simulink model "ThermalBehaviour_simulink"  (R2022a)
settings: Solver=FixedStepAuto  StartTime=0.0  StopTime=10.0  FixedStep=1  RelTol=1e-3
settings Model: Creator=Anupp  LastModifiedBy=Anupp

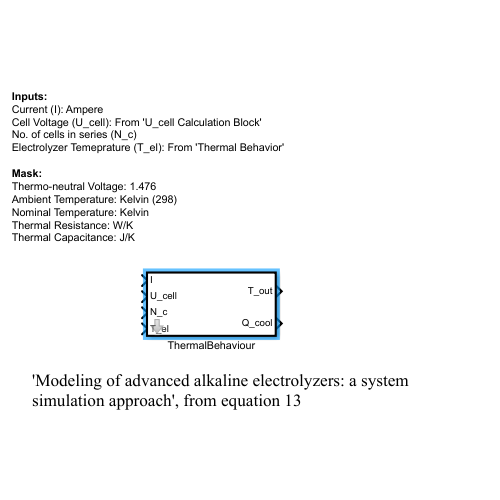
[thumbnail: Simulink's stored preview of the top-level diagram]
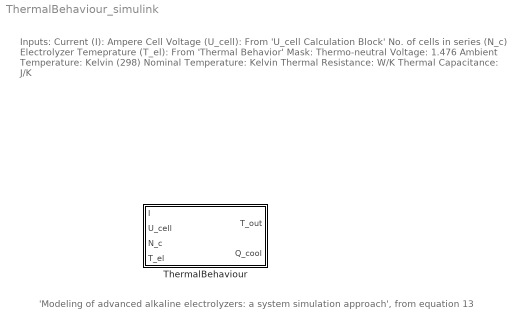
== system ThermalBehaviour_simulink ==
  note: Inputs:
      | Current (I): Ampere
      | Cell Voltage (U_cell): From 'U_cell Calculation Block'
      | No. of cells in series (N_c)
      | Electrolyzer Temeprature (T_el): From 'Thermal Behavior'
      |
      | Mask:
      | Thermo-neutral Voltage: 1.476
      | Ambient Temperature: Kelvin (298)
      | Nominal Temperature: Kelvin
      | Thermal Resistance: W/K
      | Thermal Capacitance: J/K
  note: 'Modeling of advanced alkaline electrolyzers: a system simulation approach', from equation 13
  ThermalBehaviour : Subsystem  TreatAsAtomicUnit=on  mask{E_tn=1.476, T_a=298, R_t=0, C_t=0, T_nominal=350}
      mask prompts: E_tn "Thermo-neutral voltage (E_tn)"; T_a "Ambient Temperature (kelvin)"; R_t "Thermal Resistance"; C_t "Thermal Capacitance"; T_nominal "Nominal Temperature (kelvin)"

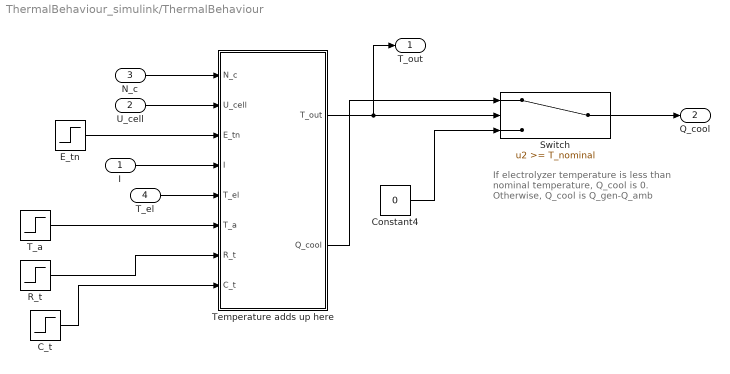
== system ThermalBehaviour_simulink/ThermalBehaviour ==
  note: If electrolyzer temperature is less than nominal temperature, Q_cool is 0.
      | Otherwise, Q_cool is Q_gen-Q_amb
  I : Inport
  U_cell : Inport  Port=2
  N_c : Inport  Port=3
  T_el : Inport  Port=4
  C_t : Step  Time=0  After=C_t  SampleTime=0
  Constant4 : Constant  Value=0
  E_tn : Step  Time=0  After=E_tn  SampleTime=0
  R_t : Step  Time=0  After=R_t  SampleTime=0
  Switch : Switch  Threshold=T_nominal  SaturateOnIntegerOverflow=off  InputSameDT=off
  T_a : Step  Time=0  After=T_a  SampleTime=0
  Temperature adds up here : Subsystem
  T_out : Outport
  Q_cool : Outport  Port=2
  wires:
  C_t/1 -> Temperature adds up here/8(C_t)
  I/1 -> Temperature adds up here/4(I)
  E_tn/1 -> Temperature adds up here/3(E_tn)
  U_cell/1 -> Temperature adds up here/2(U_cell)
  N_c/1 -> Temperature adds up here/1(N_c)
  T_a/1 -> Temperature adds up here/6(T_a)
  R_t/1 -> Temperature adds up here/7(R_t)
  T_el/1 -> Temperature adds up here/5(T_el)
  Temperature adds up here/1(T_out) -> T_out/1, Switch/2
  Constant4/1 -> Switch/3
  Switch/1 -> Q_cool/1
  Temperature adds up here/2(Q_cool) -> Switch/1

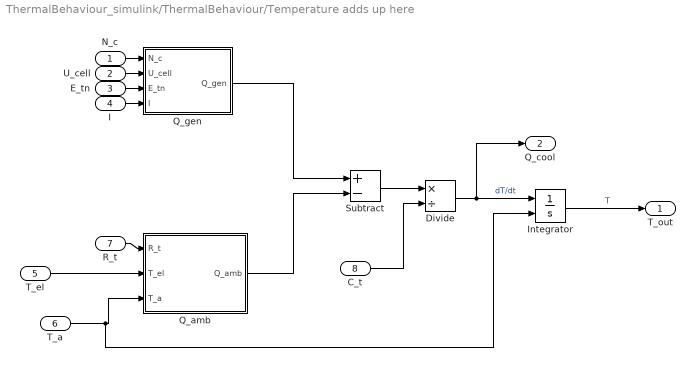
== system ThermalBehaviour_simulink/ThermalBehaviour/Temperature adds up here ==
  N_c : Inport
  U_cell : Inport  Port=2
  E_tn : Inport  Port=3
  I : Inport  Port=4
  T_el : Inport  Port=5
  T_a : Inport  Port=6
  R_t : Inport  Port=7
  C_t : Inport  Port=8
  Divide : Product  Inputs=*/
  Integrator : Integrator  InitialConditionSource=external  LimitOutput=on  UpperSaturationLimit=T_nominal
  Q_amb : MATLAB Function  TreatAsAtomicUnit=on
  Q_gen : MATLAB Function  TreatAsAtomicUnit=on
  Subtract : Sum  Inputs=+-
  T_out : Outport
  Q_cool : Outport  Port=2
  wires:
  Q_gen/1(Q_gen) -> Subtract/1
  Q_amb/1(Q_amb) -> Subtract/2
  Integrator/1 -> T_out/1  "T"
  Divide/1 -> Q_cool/1, Integrator/1  "dT/dt"
  C_t/1 -> Divide/2
  R_t/1 -> Q_amb/1(R_t)
  Subtract/1 -> Divide/1
  N_c/1 -> Q_gen/1(N_c)
  E_tn/1 -> Q_gen/3(E_tn)
  I/1 -> Q_gen/4(I)
  U_cell/1 -> Q_gen/2(U_cell)
  T_a/1 -> Integrator/2, Q_amb/3(T_a)
  T_el/1 -> Q_amb/2(T_el)

== matlab function ThermalBehaviour_simulink/ThermalBehaviour/Temperature adds up here/Q_gen ==
  data: N_c input; Q_gen output; U_cell input; E_tn input; I input
%% Inputs: 
% No. of cells in series (N_c) 
% Electrolyzer cell voltage (U_cell): V 
% Thermo-neutral voltage (E_tn): V
% Current (I): Ampere

%% Outputs:
% Generated Heat (Q_gen): Joule

%% Main Function

function Q_gen = fcn(N_c,U_cell,E_tn,I)

Q_gen = N_c * (U_cell - E_tn) * I;

end

== matlab function ThermalBehaviour_simulink/ThermalBehaviour/Temperature adds up here/Q_amb ==
  data: R_t input; Q_amb output; T_el input; T_a input
%% Inputs: 
% Thermal Resistance (R_t): W/K
% Electrolyzer Temeperatrue(T_el): Kelvin 
% Ambient Temperature(T_a): Kelvin

%% Output:
% Ambient Heat loss (Q_amb): Joule

%% Main Function

function Q_amb = fcn(R_t,T_el,T_a)

Q_amb = (T_el - T_a)/R_t;

end
